simulink model "Triboelectric"  (R2020b)
settings: Solver=ode15s  StartTime=0.0  StopTime=120  MaxStep=0.005  RelTol=1e-3
model workspace (MATLAB code in the model file):
  | sigma = 1*10^(-6);
  | S = 0.005;  %Area
  | epsp = 2.8; %epsilon_P
  | delta = 1/100000;
  | d = 1/100000;
  | epso = 8.85*10^(-12); %epsilon_0
  | Rl=100000; %Load resistance
settings Model: Creator=Barath Krishna S  LastModifiedBy=Prashant Shettigar
settings SolverCC: ZeroCrossAlgorithm=Adaptive  AlgebraicLoopSolver=LineSearch
settings DebuggingCC: IgnoredZcDiagnostic=none

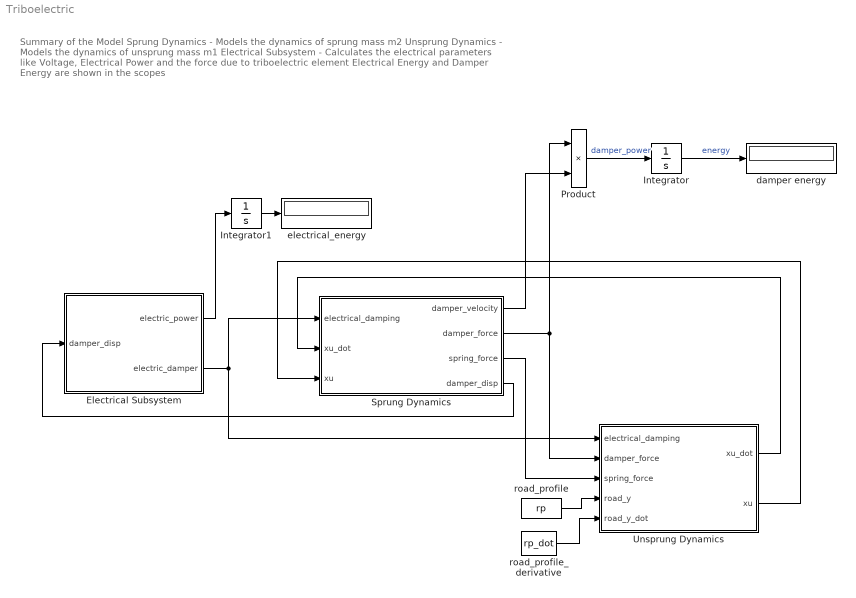
== system Triboelectric ==
  note: Summary of the Model
      | Sprung Dynamics - Models the dynamics of sprung mass m2
      | Unsprung Dynamics - Models the dynamics of unsprung mass m1
      | Electrical Subsystem - Calculates the electrical parameters like Voltage, Electrical Power and the force due to triboelectric element
      |
      | Electrical Energy and Damper Energy are shown in the scopes
  Electrical Subsystem : Subsystem
  Integrator : Integrator
  Integrator1 : Integrator
  Product : Product
  Sprung Dynamics : Subsystem
  Unsprung Dynamics : Subsystem
  damper energy : Display
      settings: Decimation=2
  electrical_energy : Display
      settings: Decimation=2
  road_profile : FromWorkspace  VariableName=rp
  road_profile_derivative : FromWorkspace  VariableName=rp_dot
  wires:
  Unsprung Dynamics/1(xu_dot) -> Sprung Dynamics/2(xu_dot)
  Unsprung Dynamics/2(xu) -> Sprung Dynamics/3(xu)
  Integrator/1 -> damper energy/1  "energy"
  road_profile/1 -> Unsprung Dynamics/4(road_y)
  Sprung Dynamics/4(damper_disp) -> Electrical Subsystem/1(damper_disp)
  road_profile_derivative/1 -> Unsprung Dynamics/5(road_y_dot)
  Sprung Dynamics/1(damper_velocity) -> Product/2
  Integrator1/1 -> electrical_energy/1
  Sprung Dynamics/3(spring_force) -> Unsprung Dynamics/3(spring_force)
  Sprung Dynamics/2(damper_force) -> Product/1, Unsprung Dynamics/2(damper_force)
  Product/1 -> Integrator/1  "damper_power"
  Electrical Subsystem/1(electric_power) -> Integrator1/1
  Electrical Subsystem/2(electric_damper) -> Unsprung Dynamics/1(electrical_damping), Sprung Dynamics/1(electrical_damping)

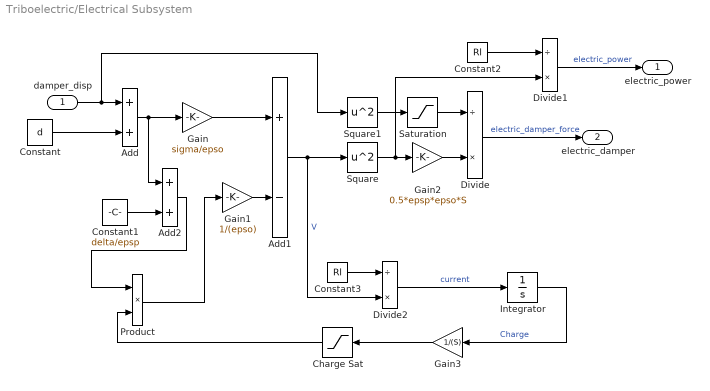
== system Triboelectric/Electrical Subsystem ==
  damper_disp : Inport
  Add : Sum
  Add1 : Sum  Inputs=+-
  Add2 : Sum
  Charge Sat : Saturate  UpperLimit=sigma  LowerLimit=0
  Constant : Constant  Value=d
  Constant1 : Constant  Value=delta/epsp
  Constant2 : Constant  Value=Rl
  Constant3 : Constant  Value=Rl
  Divide : Product  Inputs=/*
  Divide1 : Product  Inputs=/*
  Divide2 : Product  Inputs=/*
  Gain : Gain  Gain=sigma/epso
  Gain1 : Gain  Gain=1/(epso)
  Gain2 : Gain  Gain=0.5*epsp*epso*S
  Gain3 : Gain  Gain=1/(S)
  Integrator : Integrator  InitialCondition=sigma
  Product : Product
  Saturation : Saturate  UpperLimit=inf  LowerLimit=0.001
  Square : Math  Operator=square  SaturateOnIntegerOverflow=on
  Square1 : Math  Operator=square  SaturateOnIntegerOverflow=on
  electric_power : Outport
  electric_damper : Outport  Port=2
  wires:
  damper_disp/1 -> Square1/1, Add/1
  Constant/1 -> Add/2
  Add/1 -> Add2/1, Gain/1
  Gain/1 -> Add1/1
  Add2/1 -> Product/1
  Constant1/1 -> Add2/2
  Gain1/1 -> Add1/2
  Add1/1 -> Divide2/2, Square/1  "V"
  Square/1 -> Divide1/2, Gain2/1
  Gain2/1 -> Divide/2
  Square1/1 -> Saturation/1
  Divide/1 -> electric_damper/1  "electric_damper_force"
  Divide1/1 -> electric_power/1  "electric_power"
  Constant2/1 -> Divide1/1
  Saturation/1 -> Divide/1
  Constant3/1 -> Divide2/1
  Divide2/1 -> Integrator/1  "current"
  Integrator/1 -> Gain3/1  "Charge"
  Product/1 -> Gain1/1
  Gain3/1 -> Charge Sat/1
  Charge Sat/1 -> Product/2

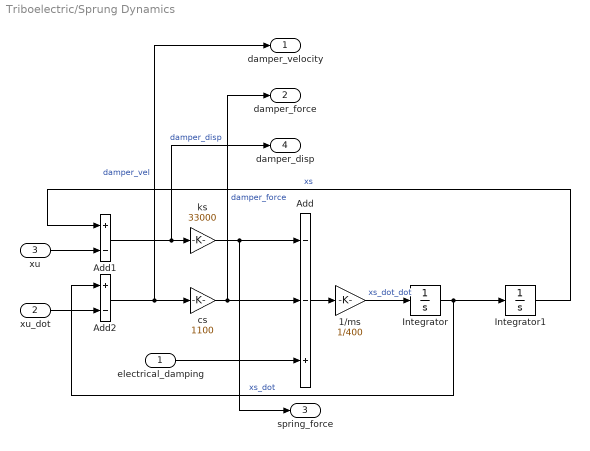
== system Triboelectric/Sprung Dynamics ==
  electrical_damping : Inport
  xu_dot : Inport  Port=2
  xu : Inport  Port=3
  1/ms : Gain  Gain=1/400
  Add : Sum  Inputs=--+
  Add1 : Sum  Inputs=+-
  Add2 : Sum  Inputs=+-
  Integrator : Integrator
  Integrator1 : Integrator
  cs : Gain  Gain=1100
  ks : Gain  Gain=33000
  damper_velocity : Outport
  damper_force : Outport  Port=2
  spring_force : Outport  Port=3
  damper_disp : Outport  Port=4
  wires:
  1/ms/1 -> Integrator/1  "xs_dot_dot"
  Add2/1 -> damper_velocity/1, cs/1  "damper_vel"
  ks/1 -> spring_force/1, Add/1
  Add/1 -> 1/ms/1
  Add1/1 -> damper_disp/1, ks/1  "damper_disp"
  Integrator1/1 -> Add1/1  "xs"
  cs/1 -> Add/2, damper_force/1  "damper_force"
  xu/1 -> Add1/2
  Integrator/1 -> Integrator1/1, Add2/1  "xs_dot"
  xu_dot/1 -> Add2/2
  electrical_damping/1 -> Add/3

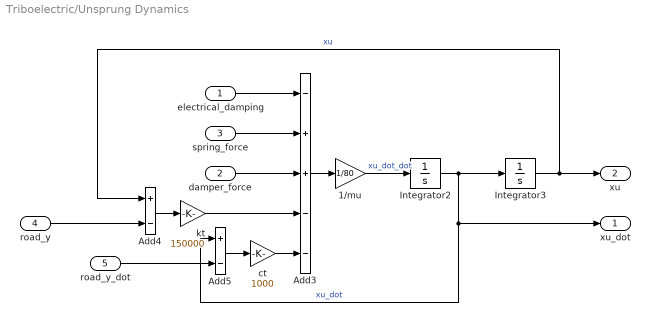
== system Triboelectric/Unsprung Dynamics ==
  electrical_damping : Inport
  damper_force : Inport  Port=2
  spring_force : Inport  Port=3
  road_y : Inport  Port=4
  road_y_dot : Inport  Port=5
  1/mu : Gain  Gain=1/80
  Add3 : Sum  Inputs=-++--
  Add4 : Sum  Inputs=+-
  Add5 : Sum  Inputs=+-
  Integrator2 : Integrator
  Integrator3 : Integrator
  ct : Gain  Gain=1000
  kt : Gain  Gain=150000
  xu_dot : Outport
  xu : Outport  Port=2
  wires:
  road_y_dot/1 -> Add5/2
  1/mu/1 -> Integrator2/1  "xu_dot_dot"
  kt/1 -> Add3/4
  ct/1 -> Add3/5
  Add3/1 -> 1/mu/1
  Add4/1 -> kt/1
  Add5/1 -> ct/1
  Integrator3/1 -> xu/1, Add4/1  "xu"
  Integrator2/1 -> xu_dot/1, Add5/1, Integrator3/1  "xu_dot"
  damper_force/1 -> Add3/3
  spring_force/1 -> Add3/2
  road_y/1 -> Add4/2
  electrical_damping/1 -> Add3/1
